simulink model "SVM_sim"  (R2018b)
settings: Solver=VariableStepAuto  StartTime=0.0  StopTime=Inf  FixedStep=T/4  RelTol=1e-3
PostLoadFcn:
  | , if any(exist('dsrtsu_mdlpostloadfcn', 'file') ~= 0), dsrtsu_mdlpostloadfcn('Execute', bdroot); end,
values from neighbouring files (symbols this model uses):
  fixed_io_gain = 175    [parameters.m]
  fixed_vclamp_gain = 1000    [parameters.m]
  fixed_vi_gain = 5800    [parameters.m]
  ioa_gain = 1    [parameters.m]
  ioa_offset = -39.67    [parameters.m]
  iob_gain = 1    [parameters.m]
  iob_offset = -40.05    [parameters.m]
  ioc_gain = 1    [parameters.m]
  ioc_offset = -39.51    [parameters.m]
  N = 500    [parameters.m]
  phi = 0    [parameters.m]
  threshold = 100    [parameters.m]
  vclamp_gain = 1    [parameters.m]
  vclamp_offset = -0.9    [parameters.m]
  via_gain = 1    [parameters.m]
  via_offset = -836.4    [parameters.m]
  vib_gain = 1    [parameters.m]
  vib_offset = -854.9    [parameters.m]
  vic_gain = 1    [parameters.m]
  vic_offset = -852.3    [parameters.m]
libraries: xbsIndex_r4 x465, rtiproclib x10, rti1202lib_adc_class1 x8, simulink x4, powerlib_meascontrol x1, rtifpgainterfacelib x1
(part 6 of 9)

== system SVM_sim/ref_generator ==
  Amp_ref : Constant  Value=5
  Constant2 : Constant  Value=2*pi/3
  Constant3 : Constant  Value=4*pi/3
  Cos : Trigonometry  Operator=cos
  Gain1 : Gain  Gain=2*pi
  Integrator : Integrator
  Multiply : Product
  Mux2 : Mux  Inputs=3
  Sum7 : Sum  Inputs=++|
  Sum8 : Sum  Inputs=++|
  f_ref : Constant  Value=50
  v_ref : Outport
  wt : Outport  Port=2
  amplitude : Outport  Port=3
  wires:
  Cos/1 -> Multiply/2
  Sum7/1 -> Mux2/2
  Sum8/1 -> Mux2/3
  Constant2/1 -> Sum7/2
  Mux2/1 -> Cos/1
  Constant3/1 -> Sum8/2
  Integrator/1 -> Sum7/1, wt/1, Sum8/1, Mux2/1
  Gain1/1 -> Integrator/1
  Multiply/1 -> v_ref/1
  f_ref/1 -> Gain1/1
  Amp_ref/1 -> amplitude/1, Multiply/1

== system SVM_sim/RTI Data/RTI Data Store ==
  RTI Data Store : Subsystem  mask(RTI_DATA_STORE){}
      mask help:
      | RTI Data Store Block. This block is used by RTI to store internal model dependent data. Deleting this block will result in data loss.
      |
      | NEVER DELETE, COPY, OR MODIFY THIS BLOCK!
      mask Help:
      | RTI Data Store Block. This block is used by RTI to store internal model dependent data. Deleting this block will result in data loss.
      | 
      | NEVER DELETE, COPY, OR MODIFY THIS BLOCK!
      mask Display: text(0.5, 0.5, ' ', 'HorizontalAlignment', 'center');

== system SVM_sim/fpga_svm/FPGA_INT_BL1 ==
  Int : Inport
  CEP1 : xbsIndex_r4/Clock Enable Probe  inherit_constraints=off  block_type=ceprobe
      settings: infoedit="Clock enable extractor.  Produces a Boolean output that mirrors the hardware clock enable associated with the input sample rate.<br><br>Hardware notes: in hardware this block costs nothing."
  Constant1 : xbsIndex_r4/Constant  const=1  gui_display_data_type=Fixed-point  arith_type=Boolean  n_bits=16  bin_pt=14  preci_type=Single  exp_width=8  frac_width=24  explicit_period=on  period=1*1e-08  equ=P=C  opselect=C  inp2=PCIN>>17  opr=+  inp1=P  carry=CIN  dbl_ovrd=off  block_type=constant
  Convert1 : xbsIndex_r4/Convert  gui_display_data_type=Fixed-point  arith_type=Unsigned  n_bits=1  bin_pt=0  float_type=Single  exp_bits=8  fraction_bits=24  quantization=Truncate  overflow=Wrap  en=off  latency=0  pipeline=off  dbl_ovrd=off  block_type=convert
  Register1 : xbsIndex_r4/Register  init=0  rst=off  en=on  dbl_ovrd=off  block_type=register
  Terminator : Terminator
  phs_interrupt : Subsystem
  usr_interrupt_00 : xbsIndex_r4/Gateway Out  inherit_from_input=off  hdl_port=on  rows=1  columns=1  UseAsDAC=off  DACChannel='1'  interface=None  automatic_assignment=on  address_offset=hex2dec('00')  intf_name=''  intf_description=''  timing_constraint=None  locs_specified=off  LOCs={}  io_standard={}  block_type=gatewayout
  tag scope: CN_SVM_sim_1_read_Interrupt_1_data_o=global
  wires:
  Constant1/1 -> CEP1/1
  CEP1/1 -> Register1/2
  Register1/1 -> usr_interrupt_00/1
  Int/1 -> Convert1/1
  Convert1/1 -> Register1/1
  usr_interrupt_00/1 -> phs_interrupt/1(data_i)
  phs_interrupt/1(data_o) -> [CN_SVM_sim_1_read_Interrupt_1_data_o], Terminator/1

== system SVM_sim/fpga_svm/FPGA_INT_BL2 ==
  Int : Inport
  CEP1 : xbsIndex_r4/Clock Enable Probe  inherit_constraints=off  block_type=ceprobe
      settings: infoedit="Clock enable extractor.  Produces a Boolean output that mirrors the hardware clock enable associated with the input sample rate.<br><br>Hardware notes: in hardware this block costs nothing."
  Constant1 : xbsIndex_r4/Constant  const=1  gui_display_data_type=Fixed-point  arith_type=Boolean  n_bits=16  bin_pt=14  preci_type=Single  exp_width=8  frac_width=24  explicit_period=on  period=1*1e-08  equ=P=C  opselect=C  inp2=PCIN>>17  opr=+  inp1=P  carry=CIN  dbl_ovrd=off  block_type=constant
  Convert1 : xbsIndex_r4/Convert  gui_display_data_type=Fixed-point  arith_type=Unsigned  n_bits=1  bin_pt=0  float_type=Single  exp_bits=8  fraction_bits=24  quantization=Truncate  overflow=Wrap  en=off  latency=0  pipeline=off  dbl_ovrd=off  block_type=convert
  Register1 : xbsIndex_r4/Register  init=0  rst=off  en=on  dbl_ovrd=off  block_type=register
  Terminator : Terminator
  phs_interrupt : Subsystem
  usr_interrupt_01 : xbsIndex_r4/Gateway Out  inherit_from_input=off  hdl_port=on  rows=1  columns=1  UseAsDAC=off  DACChannel='1'  interface=None  automatic_assignment=on  address_offset=hex2dec('00')  intf_name=''  intf_description=''  timing_constraint=None  locs_specified=off  LOCs={}  io_standard={}  block_type=gatewayout
  tag scope: CN_SVM_sim_1_read_Interrupt_2_data_o=global
  wires:
  Constant1/1 -> CEP1/1
  CEP1/1 -> Register1/2
  Register1/1 -> usr_interrupt_01/1
  Int/1 -> Convert1/1
  Convert1/1 -> Register1/1
  usr_interrupt_01/1 -> phs_interrupt/1(data_i)
  phs_interrupt/1(data_o) -> [CN_SVM_sim_1_read_Interrupt_2_data_o], Terminator/1

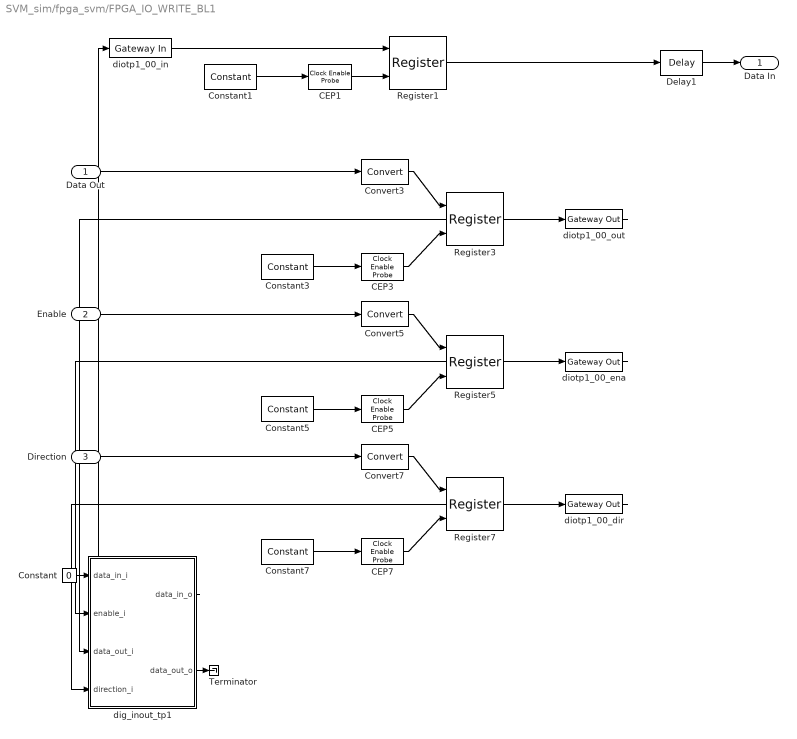
== system SVM_sim/fpga_svm/FPGA_IO_WRITE_BL1 ==
  Data Out : Inport
  Enable : Inport  Port=2
  Direction : Inport  Port=3
  CEP{1,3,5,7} (4 alike) : xbsIndex_r4/Clock Enable Probe  inherit_constraints=off  block_type=ceprobe
      settings: infoedit="Clock enable extractor.  Produces a Boolean output that mirrors the hardware clock enable associated with the input sample rate.<br><br>Hardware notes: in hardware this block costs nothing."
  Constant : Constant  Value=0
  Constant{1,3,5,7} (4 alike) : xbsIndex_r4/Constant  const=1  gui_display_data_type=Fixed-point  arith_type=Boolean  n_bits=16  bin_pt=14  preci_type=Single  exp_width=8  frac_width=24  explicit_period=on  period=1*1e-08  equ=P=C  opselect=C  inp2=PCIN>>17  opr=+  inp1=P  carry=CIN  dbl_ovrd=off  block_type=constant
  Convert3 : xbsIndex_r4/Convert  gui_display_data_type=Fixed-point  arith_type=Unsigned  n_bits=1  bin_pt=0  float_type=Single  exp_bits=8  fraction_bits=24  quantization=Truncate  overflow=Wrap  en=off  latency=0  pipeline=off  dbl_ovrd=off  block_type=convert
  Convert5 : xbsIndex_r4/Convert  gui_display_data_type=Fixed-point  arith_type=Unsigned  n_bits=1  bin_pt=0  float_type=Single  exp_bits=8  fraction_bits=24  quantization=Truncate  overflow=Wrap  en=off  latency=0  pipeline=off  dbl_ovrd=off  block_type=convert
  Convert7 : xbsIndex_r4/Convert  gui_display_data_type=Fixed-point  arith_type=Unsigned  n_bits=1  bin_pt=0  float_type=Single  exp_bits=8  fraction_bits=24  quantization=Truncate  overflow=Wrap  en=off  latency=0  pipeline=off  dbl_ovrd=off  block_type=convert
  Delay1 : xbsIndex_r4/Delay  rst=off  infoeditControl=Selection of Reset will increase slice count due to use of real FFs and instead of SRLs  en=off  latency=0  reg_retiming=off  dbl_ovrd=off  block_type=delay
  Register{1,3,5,7} (4 alike) : xbsIndex_r4/Register  init=0  rst=off  en=on  dbl_ovrd=off  block_type=register
  Terminator : Terminator
  dig_inout_tp1 : Subsystem
      mask init:
      | par = rtifpgafcnlib('GetCurrentParaValue', get_param(get(gcbh, 'parent'), 'handle'));
      | inverted_dio = str2double(par(2).Value{1});
      | vsetting = str2double(par(5).Value{1});
      | switch vsetting 
      |     case 1
      |         voltage = 3.3
      |     case 2
      |         voltage = 2.5;
      |     otherwise
      |         voltage = 5;
      | end
  diotp1_00_dir : xbsIndex_r4/Gateway Out  inherit_from_input=off  hdl_port=on  rows=1  columns=1  UseAsDAC=off  DACChannel='1'  interface=None  automatic_assignment=on  address_offset=hex2dec('00')  intf_name=''  intf_description=''  timing_constraint=None  locs_specified=off  LOCs={}  io_standard={}  block_type=gatewayout
  diotp1_00_ena : xbsIndex_r4/Gateway Out  inherit_from_input=off  hdl_port=on  rows=1  columns=1  UseAsDAC=off  DACChannel='1'  interface=None  automatic_assignment=on  address_offset=hex2dec('00')  intf_name=''  intf_description=''  timing_constraint=None  locs_specified=off  LOCs={}  io_standard={}  block_type=gatewayout
  diotp1_00_in : xbsIndex_r4/Gateway In  gui_display_data_type=Fixed-point  arith_type=Unsigned  n_bits=1  bin_pt=0  preci_type=Single  exp_width=8  frac_width=24  rows=1  columns=1  quantization="Round  (unbiased: +/- Inf)"  overflow=Saturate  period=1e-08  UseAsADC=off  ADCChannel='1'  interface=None  automatic_assignment=on  address_offset=hex2dec('00')  intf_name=''  intf_description=''  default_value=0  timing_constraint=None  locs_specified=off  LOCs={}  io_standard={}  inherit_from_input=off  hdl_port=on  dbl_ovrd=off  block_type=gatewayin
  diotp1_00_out : xbsIndex_r4/Gateway Out  inherit_from_input=off  hdl_port=on  rows=1  columns=1  UseAsDAC=off  DACChannel='1'  interface=None  automatic_assignment=on  address_offset=hex2dec('00')  intf_name=''  intf_description=''  timing_constraint=None  locs_specified=off  LOCs={}  io_standard={}  block_type=gatewayout
  Data In : Outport
  wires:
  Register1/1 -> Delay1/1
  Delay1/1 -> Data In/1
  Constant1/1 -> CEP1/1
  CEP1/1 -> Register1/2
  diotp1_00_in/1 -> Register1/1
  Constant3/1 -> CEP3/1
  CEP3/1 -> Register3/2
  Register3/1 -> diotp1_00_out/1
  Data Out/1 -> Convert3/1
  Convert3/1 -> Register3/1
  Constant5/1 -> CEP5/1
  CEP5/1 -> Register5/2
  Register5/1 -> diotp1_00_ena/1
  Enable/1 -> Convert5/1
  Convert5/1 -> Register5/1
  Constant7/1 -> CEP7/1
  CEP7/1 -> Register7/2
  Register7/1 -> diotp1_00_dir/1
  Direction/1 -> Convert7/1
  Convert7/1 -> Register7/1
  dig_inout_tp1/1(data_in_o) -> diotp1_00_in/1
  diotp1_00_out/1 -> dig_inout_tp1/3(data_out_i)
  diotp1_00_ena/1 -> dig_inout_tp1/2(enable_i)
  diotp1_00_dir/1 -> dig_inout_tp1/4(direction_i)
  Constant/1 -> dig_inout_tp1/1(data_in_i)
  dig_inout_tp1/2(data_out_o) -> Terminator/1

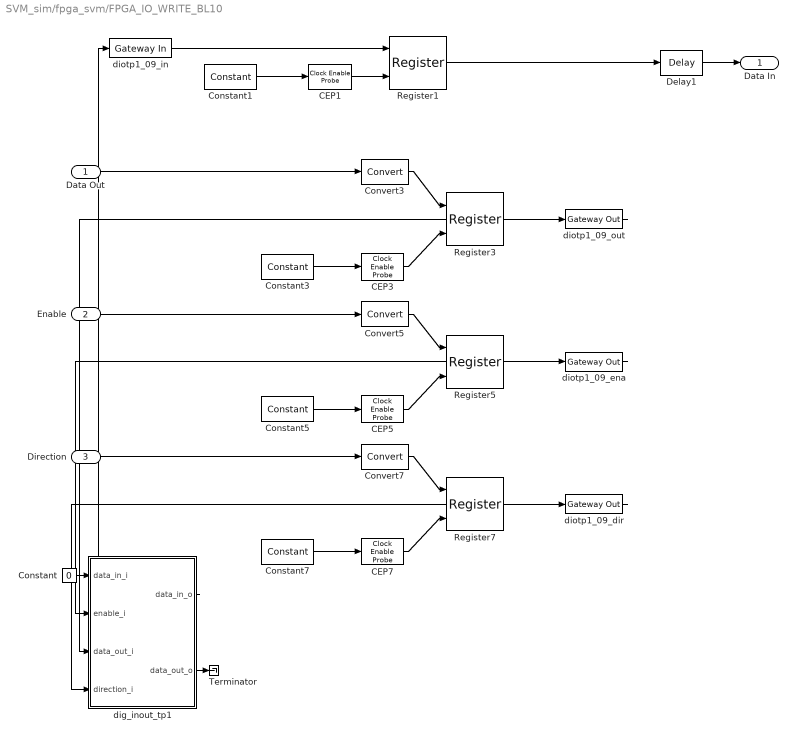
== system SVM_sim/fpga_svm/FPGA_IO_WRITE_BL10 ==
  Data Out : Inport
  Enable : Inport  Port=2
  Direction : Inport  Port=3
  CEP{1,3,5,7} (4 alike) : xbsIndex_r4/Clock Enable Probe  inherit_constraints=off  block_type=ceprobe
      settings: infoedit="Clock enable extractor.  Produces a Boolean output that mirrors the hardware clock enable associated with the input sample rate.<br><br>Hardware notes: in hardware this block costs nothing."
  Constant : Constant  Value=0
  Constant{1,3,5,7} (4 alike) : xbsIndex_r4/Constant  const=1  gui_display_data_type=Fixed-point  arith_type=Boolean  n_bits=16  bin_pt=14  preci_type=Single  exp_width=8  frac_width=24  explicit_period=on  period=1*1e-08  equ=P=C  opselect=C  inp2=PCIN>>17  opr=+  inp1=P  carry=CIN  dbl_ovrd=off  block_type=constant
  Convert3 : xbsIndex_r4/Convert  gui_display_data_type=Fixed-point  arith_type=Unsigned  n_bits=1  bin_pt=0  float_type=Single  exp_bits=8  fraction_bits=24  quantization=Truncate  overflow=Wrap  en=off  latency=0  pipeline=off  dbl_ovrd=off  block_type=convert
  Convert5 : xbsIndex_r4/Convert  gui_display_data_type=Fixed-point  arith_type=Unsigned  n_bits=1  bin_pt=0  float_type=Single  exp_bits=8  fraction_bits=24  quantization=Truncate  overflow=Wrap  en=off  latency=0  pipeline=off  dbl_ovrd=off  block_type=convert
  Convert7 : xbsIndex_r4/Convert  gui_display_data_type=Fixed-point  arith_type=Unsigned  n_bits=1  bin_pt=0  float_type=Single  exp_bits=8  fraction_bits=24  quantization=Truncate  overflow=Wrap  en=off  latency=0  pipeline=off  dbl_ovrd=off  block_type=convert
  Delay1 : xbsIndex_r4/Delay  rst=off  infoeditControl=Selection of Reset will increase slice count due to use of real FFs and instead of SRLs  en=off  latency=0  reg_retiming=off  dbl_ovrd=off  block_type=delay
  Register{1,3,5,7} (4 alike) : xbsIndex_r4/Register  init=0  rst=off  en=on  dbl_ovrd=off  block_type=register
  Terminator : Terminator
  dig_inout_tp1 : Subsystem
      mask init: same as SVM_sim/fpga_svm/FPGA_IO_WRITE_BL1/dig_inout_tp1
  diotp1_09_dir : xbsIndex_r4/Gateway Out  inherit_from_input=off  hdl_port=on  rows=1  columns=1  UseAsDAC=off  DACChannel='1'  interface=None  automatic_assignment=on  address_offset=hex2dec('00')  intf_name=''  intf_description=''  timing_constraint=None  locs_specified=off  LOCs={}  io_standard={}  block_type=gatewayout
  diotp1_09_ena : xbsIndex_r4/Gateway Out  inherit_from_input=off  hdl_port=on  rows=1  columns=1  UseAsDAC=off  DACChannel='1'  interface=None  automatic_assignment=on  address_offset=hex2dec('00')  intf_name=''  intf_description=''  timing_constraint=None  locs_specified=off  LOCs={}  io_standard={}  block_type=gatewayout
  diotp1_09_in : xbsIndex_r4/Gateway In  gui_display_data_type=Fixed-point  arith_type=Unsigned  n_bits=1  bin_pt=0  preci_type=Single  exp_width=8  frac_width=24  rows=1  columns=1  quantization="Round  (unbiased: +/- Inf)"  overflow=Saturate  period=1e-08  UseAsADC=off  ADCChannel='1'  interface=None  automatic_assignment=on  address_offset=hex2dec('00')  intf_name=''  intf_description=''  default_value=0  timing_constraint=None  locs_specified=off  LOCs={}  io_standard={}  inherit_from_input=off  hdl_port=on  dbl_ovrd=off  block_type=gatewayin
  diotp1_09_out : xbsIndex_r4/Gateway Out  inherit_from_input=off  hdl_port=on  rows=1  columns=1  UseAsDAC=off  DACChannel='1'  interface=None  automatic_assignment=on  address_offset=hex2dec('00')  intf_name=''  intf_description=''  timing_constraint=None  locs_specified=off  LOCs={}  io_standard={}  block_type=gatewayout
  Data In : Outport
  wires:
  Register1/1 -> Delay1/1
  Delay1/1 -> Data In/1
  Constant1/1 -> CEP1/1
  CEP1/1 -> Register1/2
  diotp1_09_in/1 -> Register1/1
  Constant3/1 -> CEP3/1
  CEP3/1 -> Register3/2
  Register3/1 -> diotp1_09_out/1
  Data Out/1 -> Convert3/1
  Convert3/1 -> Register3/1
  Constant5/1 -> CEP5/1
  CEP5/1 -> Register5/2
  Register5/1 -> diotp1_09_ena/1
  Enable/1 -> Convert5/1
  Convert5/1 -> Register5/1
  Constant7/1 -> CEP7/1
  CEP7/1 -> Register7/2
  Register7/1 -> diotp1_09_dir/1
  Direction/1 -> Convert7/1
  Convert7/1 -> Register7/1
  dig_inout_tp1/1(data_in_o) -> diotp1_09_in/1
  diotp1_09_out/1 -> dig_inout_tp1/3(data_out_i)
  diotp1_09_ena/1 -> dig_inout_tp1/2(enable_i)
  diotp1_09_dir/1 -> dig_inout_tp1/4(direction_i)
  Constant/1 -> dig_inout_tp1/1(data_in_i)
  dig_inout_tp1/2(data_out_o) -> Terminator/1

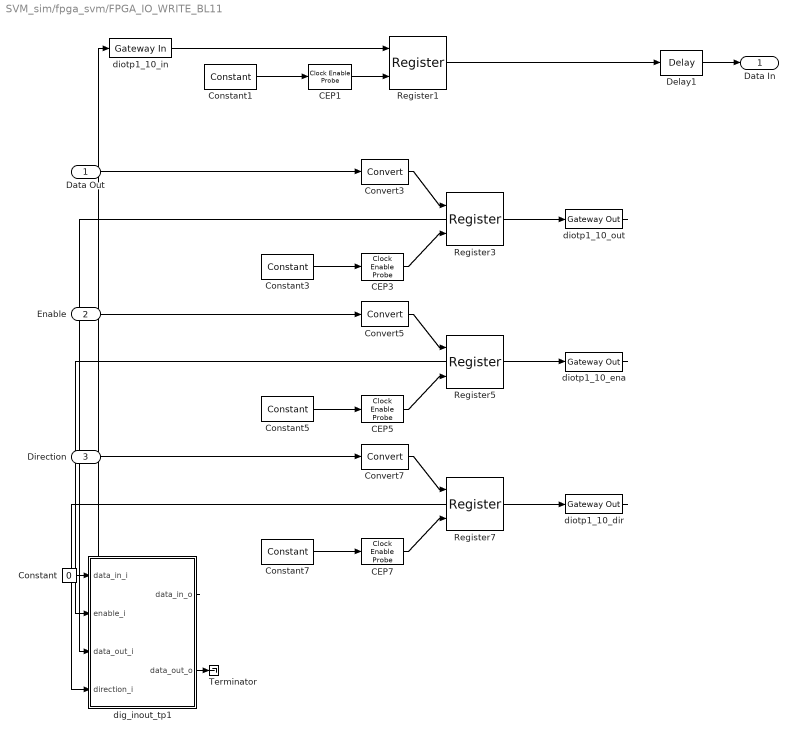
== system SVM_sim/fpga_svm/FPGA_IO_WRITE_BL11 ==
  Data Out : Inport
  Enable : Inport  Port=2
  Direction : Inport  Port=3
  CEP{1,3,5,7} (4 alike) : xbsIndex_r4/Clock Enable Probe  inherit_constraints=off  block_type=ceprobe
      settings: infoedit="Clock enable extractor.  Produces a Boolean output that mirrors the hardware clock enable associated with the input sample rate.<br><br>Hardware notes: in hardware this block costs nothing."
  Constant : Constant  Value=0
  Constant{1,3,5,7} (4 alike) : xbsIndex_r4/Constant  const=1  gui_display_data_type=Fixed-point  arith_type=Boolean  n_bits=16  bin_pt=14  preci_type=Single  exp_width=8  frac_width=24  explicit_period=on  period=1*1e-08  equ=P=C  opselect=C  inp2=PCIN>>17  opr=+  inp1=P  carry=CIN  dbl_ovrd=off  block_type=constant
  Convert3 : xbsIndex_r4/Convert  gui_display_data_type=Fixed-point  arith_type=Unsigned  n_bits=1  bin_pt=0  float_type=Single  exp_bits=8  fraction_bits=24  quantization=Truncate  overflow=Wrap  en=off  latency=0  pipeline=off  dbl_ovrd=off  block_type=convert
  Convert5 : xbsIndex_r4/Convert  gui_display_data_type=Fixed-point  arith_type=Unsigned  n_bits=1  bin_pt=0  float_type=Single  exp_bits=8  fraction_bits=24  quantization=Truncate  overflow=Wrap  en=off  latency=0  pipeline=off  dbl_ovrd=off  block_type=convert
  Convert7 : xbsIndex_r4/Convert  gui_display_data_type=Fixed-point  arith_type=Unsigned  n_bits=1  bin_pt=0  float_type=Single  exp_bits=8  fraction_bits=24  quantization=Truncate  overflow=Wrap  en=off  latency=0  pipeline=off  dbl_ovrd=off  block_type=convert
  Delay1 : xbsIndex_r4/Delay  rst=off  infoeditControl=Selection of Reset will increase slice count due to use of real FFs and instead of SRLs  en=off  latency=0  reg_retiming=off  dbl_ovrd=off  block_type=delay
  Register{1,3,5,7} (4 alike) : xbsIndex_r4/Register  init=0  rst=off  en=on  dbl_ovrd=off  block_type=register
  Terminator : Terminator
  dig_inout_tp1 : Subsystem
      mask init: same as SVM_sim/fpga_svm/FPGA_IO_WRITE_BL1/dig_inout_tp1
  diotp1_10_dir : xbsIndex_r4/Gateway Out  inherit_from_input=off  hdl_port=on  rows=1  columns=1  UseAsDAC=off  DACChannel='1'  interface=None  automatic_assignment=on  address_offset=hex2dec('00')  intf_name=''  intf_description=''  timing_constraint=None  locs_specified=off  LOCs={}  io_standard={}  block_type=gatewayout
  diotp1_10_ena : xbsIndex_r4/Gateway Out  inherit_from_input=off  hdl_port=on  rows=1  columns=1  UseAsDAC=off  DACChannel='1'  interface=None  automatic_assignment=on  address_offset=hex2dec('00')  intf_name=''  intf_description=''  timing_constraint=None  locs_specified=off  LOCs={}  io_standard={}  block_type=gatewayout
  diotp1_10_in : xbsIndex_r4/Gateway In  gui_display_data_type=Fixed-point  arith_type=Unsigned  n_bits=1  bin_pt=0  preci_type=Single  exp_width=8  frac_width=24  rows=1  columns=1  quantization="Round  (unbiased: +/- Inf)"  overflow=Saturate  period=1e-08  UseAsADC=off  ADCChannel='1'  interface=None  automatic_assignment=on  address_offset=hex2dec('00')  intf_name=''  intf_description=''  default_value=0  timing_constraint=None  locs_specified=off  LOCs={}  io_standard={}  inherit_from_input=off  hdl_port=on  dbl_ovrd=off  block_type=gatewayin
  diotp1_10_out : xbsIndex_r4/Gateway Out  inherit_from_input=off  hdl_port=on  rows=1  columns=1  UseAsDAC=off  DACChannel='1'  interface=None  automatic_assignment=on  address_offset=hex2dec('00')  intf_name=''  intf_description=''  timing_constraint=None  locs_specified=off  LOCs={}  io_standard={}  block_type=gatewayout
  Data In : Outport
  wires:
  Register1/1 -> Delay1/1
  Delay1/1 -> Data In/1
  Constant1/1 -> CEP1/1
  CEP1/1 -> Register1/2
  diotp1_10_in/1 -> Register1/1
  Constant3/1 -> CEP3/1
  CEP3/1 -> Register3/2
  Register3/1 -> diotp1_10_out/1
  Data Out/1 -> Convert3/1
  Convert3/1 -> Register3/1
  Constant5/1 -> CEP5/1
  CEP5/1 -> Register5/2
  Register5/1 -> diotp1_10_ena/1
  Enable/1 -> Convert5/1
  Convert5/1 -> Register5/1
  Constant7/1 -> CEP7/1
  CEP7/1 -> Register7/2
  Register7/1 -> diotp1_10_dir/1
  Direction/1 -> Convert7/1
  Convert7/1 -> Register7/1
  dig_inout_tp1/1(data_in_o) -> diotp1_10_in/1
  diotp1_10_out/1 -> dig_inout_tp1/3(data_out_i)
  diotp1_10_ena/1 -> dig_inout_tp1/2(enable_i)
  diotp1_10_dir/1 -> dig_inout_tp1/4(direction_i)
  Constant/1 -> dig_inout_tp1/1(data_in_i)
  dig_inout_tp1/2(data_out_o) -> Terminator/1

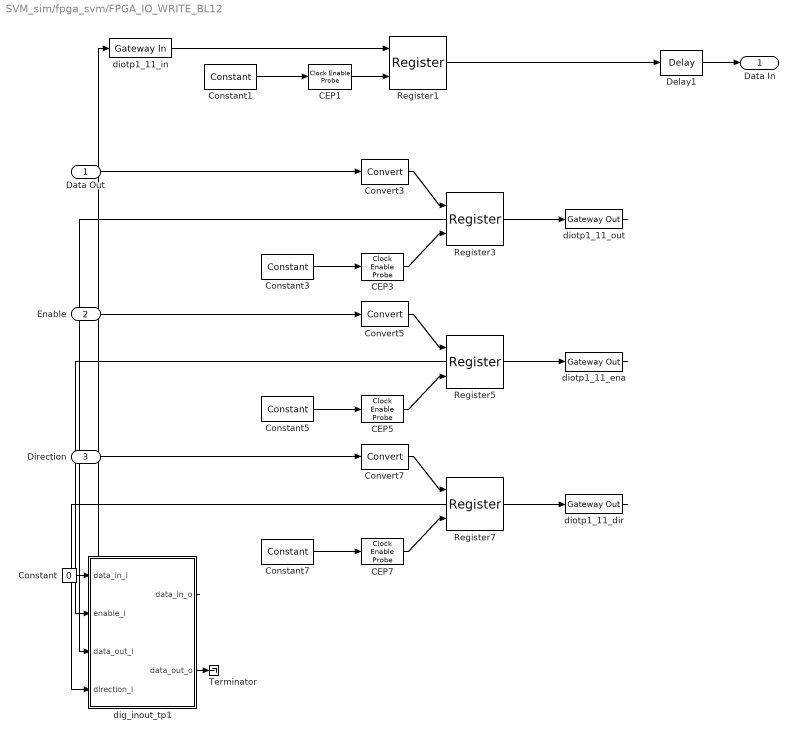
== system SVM_sim/fpga_svm/FPGA_IO_WRITE_BL12 ==
  Data Out : Inport
  Enable : Inport  Port=2
  Direction : Inport  Port=3
  CEP{1,3,5,7} (4 alike) : xbsIndex_r4/Clock Enable Probe  inherit_constraints=off  block_type=ceprobe
      settings: infoedit="Clock enable extractor.  Produces a Boolean output that mirrors the hardware clock enable associated with the input sample rate.<br><br>Hardware notes: in hardware this block costs nothing."
  Constant : Constant  Value=0
  Constant{1,3,5,7} (4 alike) : xbsIndex_r4/Constant  const=1  gui_display_data_type=Fixed-point  arith_type=Boolean  n_bits=16  bin_pt=14  preci_type=Single  exp_width=8  frac_width=24  explicit_period=on  period=1*1e-08  equ=P=C  opselect=C  inp2=PCIN>>17  opr=+  inp1=P  carry=CIN  dbl_ovrd=off  block_type=constant
  Convert3 : xbsIndex_r4/Convert  gui_display_data_type=Fixed-point  arith_type=Unsigned  n_bits=1  bin_pt=0  float_type=Single  exp_bits=8  fraction_bits=24  quantization=Truncate  overflow=Wrap  en=off  latency=0  pipeline=off  dbl_ovrd=off  block_type=convert
  Convert5 : xbsIndex_r4/Convert  gui_display_data_type=Fixed-point  arith_type=Unsigned  n_bits=1  bin_pt=0  float_type=Single  exp_bits=8  fraction_bits=24  quantization=Truncate  overflow=Wrap  en=off  latency=0  pipeline=off  dbl_ovrd=off  block_type=convert
  Convert7 : xbsIndex_r4/Convert  gui_display_data_type=Fixed-point  arith_type=Unsigned  n_bits=1  bin_pt=0  float_type=Single  exp_bits=8  fraction_bits=24  quantization=Truncate  overflow=Wrap  en=off  latency=0  pipeline=off  dbl_ovrd=off  block_type=convert
  Delay1 : xbsIndex_r4/Delay  rst=off  infoeditControl=Selection of Reset will increase slice count due to use of real FFs and instead of SRLs  en=off  latency=0  reg_retiming=off  dbl_ovrd=off  block_type=delay
  Register{1,3,5,7} (4 alike) : xbsIndex_r4/Register  init=0  rst=off  en=on  dbl_ovrd=off  block_type=register
  Terminator : Terminator
  dig_inout_tp1 : Subsystem
      mask init: same as SVM_sim/fpga_svm/FPGA_IO_WRITE_BL1/dig_inout_tp1
  diotp1_11_dir : xbsIndex_r4/Gateway Out  inherit_from_input=off  hdl_port=on  rows=1  columns=1  UseAsDAC=off  DACChannel='1'  interface=None  automatic_assignment=on  address_offset=hex2dec('00')  intf_name=''  intf_description=''  timing_constraint=None  locs_specified=off  LOCs={}  io_standard={}  block_type=gatewayout
  diotp1_11_ena : xbsIndex_r4/Gateway Out  inherit_from_input=off  hdl_port=on  rows=1  columns=1  UseAsDAC=off  DACChannel='1'  interface=None  automatic_assignment=on  address_offset=hex2dec('00')  intf_name=''  intf_description=''  timing_constraint=None  locs_specified=off  LOCs={}  io_standard={}  block_type=gatewayout
  diotp1_11_in : xbsIndex_r4/Gateway In  gui_display_data_type=Fixed-point  arith_type=Unsigned  n_bits=1  bin_pt=0  preci_type=Single  exp_width=8  frac_width=24  rows=1  columns=1  quantization="Round  (unbiased: +/- Inf)"  overflow=Saturate  period=1e-08  UseAsADC=off  ADCChannel='1'  interface=None  automatic_assignment=on  address_offset=hex2dec('00')  intf_name=''  intf_description=''  default_value=0  timing_constraint=None  locs_specified=off  LOCs={}  io_standard={}  inherit_from_input=off  hdl_port=on  dbl_ovrd=off  block_type=gatewayin
  diotp1_11_out : xbsIndex_r4/Gateway Out  inherit_from_input=off  hdl_port=on  rows=1  columns=1  UseAsDAC=off  DACChannel='1'  interface=None  automatic_assignment=on  address_offset=hex2dec('00')  intf_name=''  intf_description=''  timing_constraint=None  locs_specified=off  LOCs={}  io_standard={}  block_type=gatewayout
  Data In : Outport
  wires:
  Register1/1 -> Delay1/1
  Delay1/1 -> Data In/1
  Constant1/1 -> CEP1/1
  CEP1/1 -> Register1/2
  diotp1_11_in/1 -> Register1/1
  Constant3/1 -> CEP3/1
  CEP3/1 -> Register3/2
  Register3/1 -> diotp1_11_out/1
  Data Out/1 -> Convert3/1
  Convert3/1 -> Register3/1
  Constant5/1 -> CEP5/1
  CEP5/1 -> Register5/2
  Register5/1 -> diotp1_11_ena/1
  Enable/1 -> Convert5/1
  Convert5/1 -> Register5/1
  Constant7/1 -> CEP7/1
  CEP7/1 -> Register7/2
  Register7/1 -> diotp1_11_dir/1
  Direction/1 -> Convert7/1
  Convert7/1 -> Register7/1
  dig_inout_tp1/1(data_in_o) -> diotp1_11_in/1
  diotp1_11_out/1 -> dig_inout_tp1/3(data_out_i)
  diotp1_11_ena/1 -> dig_inout_tp1/2(enable_i)
  diotp1_11_dir/1 -> dig_inout_tp1/4(direction_i)
  Constant/1 -> dig_inout_tp1/1(data_in_i)
  dig_inout_tp1/2(data_out_o) -> Terminator/1

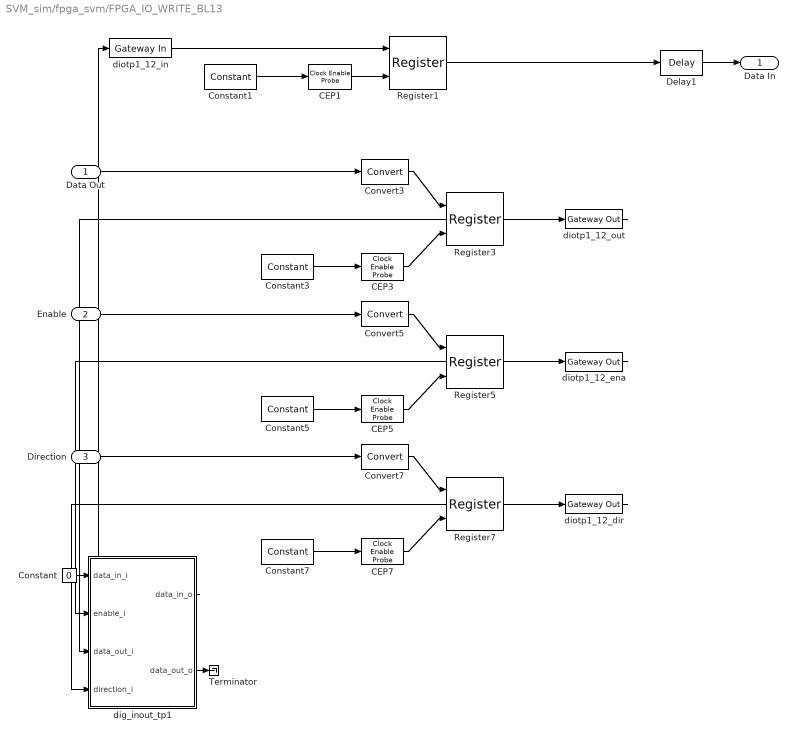
== system SVM_sim/fpga_svm/FPGA_IO_WRITE_BL13 ==
  Data Out : Inport
  Enable : Inport  Port=2
  Direction : Inport  Port=3
  CEP{1,3,5,7} (4 alike) : xbsIndex_r4/Clock Enable Probe  inherit_constraints=off  block_type=ceprobe
      settings: infoedit="Clock enable extractor.  Produces a Boolean output that mirrors the hardware clock enable associated with the input sample rate.<br><br>Hardware notes: in hardware this block costs nothing."
  Constant : Constant  Value=0
  Constant{1,3,5,7} (4 alike) : xbsIndex_r4/Constant  const=1  gui_display_data_type=Fixed-point  arith_type=Boolean  n_bits=16  bin_pt=14  preci_type=Single  exp_width=8  frac_width=24  explicit_period=on  period=1*1e-08  equ=P=C  opselect=C  inp2=PCIN>>17  opr=+  inp1=P  carry=CIN  dbl_ovrd=off  block_type=constant
  Convert3 : xbsIndex_r4/Convert  gui_display_data_type=Fixed-point  arith_type=Unsigned  n_bits=1  bin_pt=0  float_type=Single  exp_bits=8  fraction_bits=24  quantization=Truncate  overflow=Wrap  en=off  latency=0  pipeline=off  dbl_ovrd=off  block_type=convert
  Convert5 : xbsIndex_r4/Convert  gui_display_data_type=Fixed-point  arith_type=Unsigned  n_bits=1  bin_pt=0  float_type=Single  exp_bits=8  fraction_bits=24  quantization=Truncate  overflow=Wrap  en=off  latency=0  pipeline=off  dbl_ovrd=off  block_type=convert
  Convert7 : xbsIndex_r4/Convert  gui_display_data_type=Fixed-point  arith_type=Unsigned  n_bits=1  bin_pt=0  float_type=Single  exp_bits=8  fraction_bits=24  quantization=Truncate  overflow=Wrap  en=off  latency=0  pipeline=off  dbl_ovrd=off  block_type=convert
  Delay1 : xbsIndex_r4/Delay  rst=off  infoeditControl=Selection of Reset will increase slice count due to use of real FFs and instead of SRLs  en=off  latency=0  reg_retiming=off  dbl_ovrd=off  block_type=delay
  Register{1,3,5,7} (4 alike) : xbsIndex_r4/Register  init=0  rst=off  en=on  dbl_ovrd=off  block_type=register
  Terminator : Terminator
  dig_inout_tp1 : Subsystem
      mask init: same as SVM_sim/fpga_svm/FPGA_IO_WRITE_BL1/dig_inout_tp1
  diotp1_12_dir : xbsIndex_r4/Gateway Out  inherit_from_input=off  hdl_port=on  rows=1  columns=1  UseAsDAC=off  DACChannel='1'  interface=None  automatic_assignment=on  address_offset=hex2dec('00')  intf_name=''  intf_description=''  timing_constraint=None  locs_specified=off  LOCs={}  io_standard={}  block_type=gatewayout
  diotp1_12_ena : xbsIndex_r4/Gateway Out  inherit_from_input=off  hdl_port=on  rows=1  columns=1  UseAsDAC=off  DACChannel='1'  interface=None  automatic_assignment=on  address_offset=hex2dec('00')  intf_name=''  intf_description=''  timing_constraint=None  locs_specified=off  LOCs={}  io_standard={}  block_type=gatewayout
  diotp1_12_in : xbsIndex_r4/Gateway In  gui_display_data_type=Fixed-point  arith_type=Unsigned  n_bits=1  bin_pt=0  preci_type=Single  exp_width=8  frac_width=24  rows=1  columns=1  quantization="Round  (unbiased: +/- Inf)"  overflow=Saturate  period=1e-08  UseAsADC=off  ADCChannel='1'  interface=None  automatic_assignment=on  address_offset=hex2dec('00')  intf_name=''  intf_description=''  default_value=0  timing_constraint=None  locs_specified=off  LOCs={}  io_standard={}  inherit_from_input=off  hdl_port=on  dbl_ovrd=off  block_type=gatewayin
  diotp1_12_out : xbsIndex_r4/Gateway Out  inherit_from_input=off  hdl_port=on  rows=1  columns=1  UseAsDAC=off  DACChannel='1'  interface=None  automatic_assignment=on  address_offset=hex2dec('00')  intf_name=''  intf_description=''  timing_constraint=None  locs_specified=off  LOCs={}  io_standard={}  block_type=gatewayout
  Data In : Outport
  wires:
  Register1/1 -> Delay1/1
  Delay1/1 -> Data In/1
  Constant1/1 -> CEP1/1
  CEP1/1 -> Register1/2
  diotp1_12_in/1 -> Register1/1
  Constant3/1 -> CEP3/1
  CEP3/1 -> Register3/2
  Register3/1 -> diotp1_12_out/1
  Data Out/1 -> Convert3/1
  Convert3/1 -> Register3/1
  Constant5/1 -> CEP5/1
  CEP5/1 -> Register5/2
  Register5/1 -> diotp1_12_ena/1
  Enable/1 -> Convert5/1
  Convert5/1 -> Register5/1
  Constant7/1 -> CEP7/1
  CEP7/1 -> Register7/2
  Register7/1 -> diotp1_12_dir/1
  Direction/1 -> Convert7/1
  Convert7/1 -> Register7/1
  dig_inout_tp1/1(data_in_o) -> diotp1_12_in/1
  diotp1_12_out/1 -> dig_inout_tp1/3(data_out_i)
  diotp1_12_ena/1 -> dig_inout_tp1/2(enable_i)
  diotp1_12_dir/1 -> dig_inout_tp1/4(direction_i)
  Constant/1 -> dig_inout_tp1/1(data_in_i)
  dig_inout_tp1/2(data_out_o) -> Terminator/1

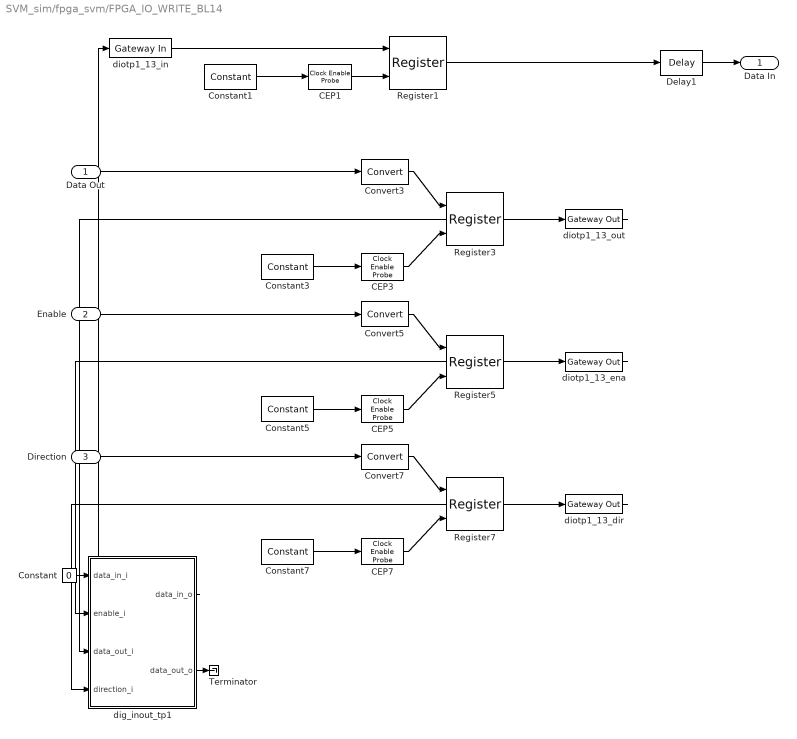
== system SVM_sim/fpga_svm/FPGA_IO_WRITE_BL14 ==
  Data Out : Inport
  Enable : Inport  Port=2
  Direction : Inport  Port=3
  CEP{1,3,5,7} (4 alike) : xbsIndex_r4/Clock Enable Probe  inherit_constraints=off  block_type=ceprobe
      settings: infoedit="Clock enable extractor.  Produces a Boolean output that mirrors the hardware clock enable associated with the input sample rate.<br><br>Hardware notes: in hardware this block costs nothing."
  Constant : Constant  Value=0
  Constant{1,3,5,7} (4 alike) : xbsIndex_r4/Constant  const=1  gui_display_data_type=Fixed-point  arith_type=Boolean  n_bits=16  bin_pt=14  preci_type=Single  exp_width=8  frac_width=24  explicit_period=on  period=1*1e-08  equ=P=C  opselect=C  inp2=PCIN>>17  opr=+  inp1=P  carry=CIN  dbl_ovrd=off  block_type=constant
  Convert3 : xbsIndex_r4/Convert  gui_display_data_type=Fixed-point  arith_type=Unsigned  n_bits=1  bin_pt=0  float_type=Single  exp_bits=8  fraction_bits=24  quantization=Truncate  overflow=Wrap  en=off  latency=0  pipeline=off  dbl_ovrd=off  block_type=convert
  Convert5 : xbsIndex_r4/Convert  gui_display_data_type=Fixed-point  arith_type=Unsigned  n_bits=1  bin_pt=0  float_type=Single  exp_bits=8  fraction_bits=24  quantization=Truncate  overflow=Wrap  en=off  latency=0  pipeline=off  dbl_ovrd=off  block_type=convert
  Convert7 : xbsIndex_r4/Convert  gui_display_data_type=Fixed-point  arith_type=Unsigned  n_bits=1  bin_pt=0  float_type=Single  exp_bits=8  fraction_bits=24  quantization=Truncate  overflow=Wrap  en=off  latency=0  pipeline=off  dbl_ovrd=off  block_type=convert
  Delay1 : xbsIndex_r4/Delay  rst=off  infoeditControl=Selection of Reset will increase slice count due to use of real FFs and instead of SRLs  en=off  latency=0  reg_retiming=off  dbl_ovrd=off  block_type=delay
  Register{1,3,5,7} (4 alike) : xbsIndex_r4/Register  init=0  rst=off  en=on  dbl_ovrd=off  block_type=register
  Terminator : Terminator
  dig_inout_tp1 : Subsystem
      mask init: same as SVM_sim/fpga_svm/FPGA_IO_WRITE_BL1/dig_inout_tp1
  diotp1_13_dir : xbsIndex_r4/Gateway Out  inherit_from_input=off  hdl_port=on  rows=1  columns=1  UseAsDAC=off  DACChannel='1'  interface=None  automatic_assignment=on  address_offset=hex2dec('00')  intf_name=''  intf_description=''  timing_constraint=None  locs_specified=off  LOCs={}  io_standard={}  block_type=gatewayout
  diotp1_13_ena : xbsIndex_r4/Gateway Out  inherit_from_input=off  hdl_port=on  rows=1  columns=1  UseAsDAC=off  DACChannel='1'  interface=None  automatic_assignment=on  address_offset=hex2dec('00')  intf_name=''  intf_description=''  timing_constraint=None  locs_specified=off  LOCs={}  io_standard={}  block_type=gatewayout
  diotp1_13_in : xbsIndex_r4/Gateway In  gui_display_data_type=Fixed-point  arith_type=Unsigned  n_bits=1  bin_pt=0  preci_type=Single  exp_width=8  frac_width=24  rows=1  columns=1  quantization="Round  (unbiased: +/- Inf)"  overflow=Saturate  period=1e-08  UseAsADC=off  ADCChannel='1'  interface=None  automatic_assignment=on  address_offset=hex2dec('00')  intf_name=''  intf_description=''  default_value=0  timing_constraint=None  locs_specified=off  LOCs={}  io_standard={}  inherit_from_input=off  hdl_port=on  dbl_ovrd=off  block_type=gatewayin
  diotp1_13_out : xbsIndex_r4/Gateway Out  inherit_from_input=off  hdl_port=on  rows=1  columns=1  UseAsDAC=off  DACChannel='1'  interface=None  automatic_assignment=on  address_offset=hex2dec('00')  intf_name=''  intf_description=''  timing_constraint=None  locs_specified=off  LOCs={}  io_standard={}  block_type=gatewayout
  Data In : Outport
  wires:
  Register1/1 -> Delay1/1
  Delay1/1 -> Data In/1
  Constant1/1 -> CEP1/1
  CEP1/1 -> Register1/2
  diotp1_13_in/1 -> Register1/1
  Constant3/1 -> CEP3/1
  CEP3/1 -> Register3/2
  Register3/1 -> diotp1_13_out/1
  Data Out/1 -> Convert3/1
  Convert3/1 -> Register3/1
  Constant5/1 -> CEP5/1
  CEP5/1 -> Register5/2
  Register5/1 -> diotp1_13_ena/1
  Enable/1 -> Convert5/1
  Convert5/1 -> Register5/1
  Constant7/1 -> CEP7/1
  CEP7/1 -> Register7/2
  Register7/1 -> diotp1_13_dir/1
  Direction/1 -> Convert7/1
  Convert7/1 -> Register7/1
  dig_inout_tp1/1(data_in_o) -> diotp1_13_in/1
  diotp1_13_out/1 -> dig_inout_tp1/3(data_out_i)
  diotp1_13_ena/1 -> dig_inout_tp1/2(enable_i)
  diotp1_13_dir/1 -> dig_inout_tp1/4(direction_i)
  Constant/1 -> dig_inout_tp1/1(data_in_i)
  dig_inout_tp1/2(data_out_o) -> Terminator/1

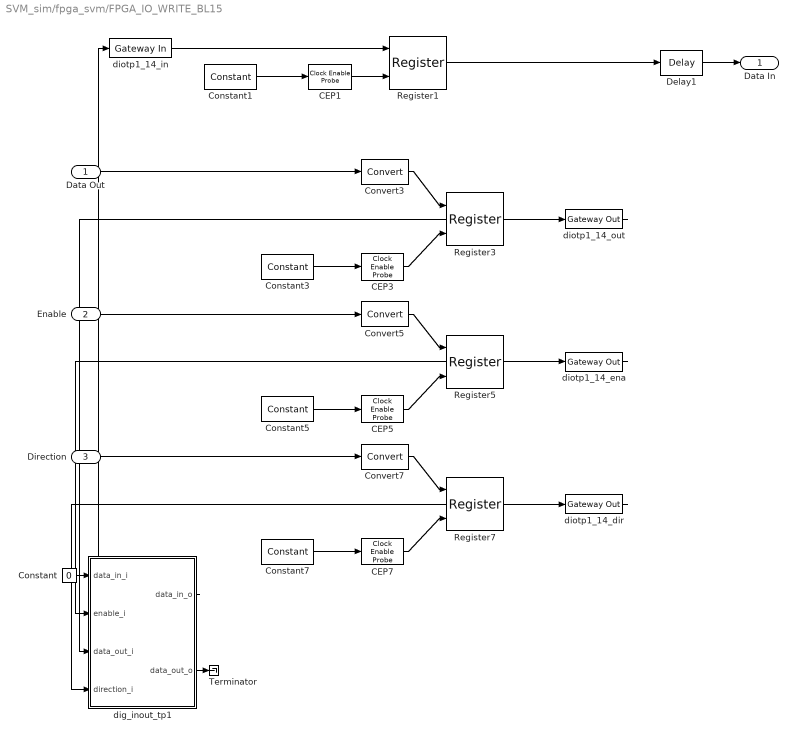
== system SVM_sim/fpga_svm/FPGA_IO_WRITE_BL15 ==
  Data Out : Inport
  Enable : Inport  Port=2
  Direction : Inport  Port=3
  CEP{1,3,5,7} (4 alike) : xbsIndex_r4/Clock Enable Probe  inherit_constraints=off  block_type=ceprobe
      settings: infoedit="Clock enable extractor.  Produces a Boolean output that mirrors the hardware clock enable associated with the input sample rate.<br><br>Hardware notes: in hardware this block costs nothing."
  Constant : Constant  Value=0
  Constant{1,3,5,7} (4 alike) : xbsIndex_r4/Constant  const=1  gui_display_data_type=Fixed-point  arith_type=Boolean  n_bits=16  bin_pt=14  preci_type=Single  exp_width=8  frac_width=24  explicit_period=on  period=1*1e-08  equ=P=C  opselect=C  inp2=PCIN>>17  opr=+  inp1=P  carry=CIN  dbl_ovrd=off  block_type=constant
  Convert3 : xbsIndex_r4/Convert  gui_display_data_type=Fixed-point  arith_type=Unsigned  n_bits=1  bin_pt=0  float_type=Single  exp_bits=8  fraction_bits=24  quantization=Truncate  overflow=Wrap  en=off  latency=0  pipeline=off  dbl_ovrd=off  block_type=convert
  Convert5 : xbsIndex_r4/Convert  gui_display_data_type=Fixed-point  arith_type=Unsigned  n_bits=1  bin_pt=0  float_type=Single  exp_bits=8  fraction_bits=24  quantization=Truncate  overflow=Wrap  en=off  latency=0  pipeline=off  dbl_ovrd=off  block_type=convert
  Convert7 : xbsIndex_r4/Convert  gui_display_data_type=Fixed-point  arith_type=Unsigned  n_bits=1  bin_pt=0  float_type=Single  exp_bits=8  fraction_bits=24  quantization=Truncate  overflow=Wrap  en=off  latency=0  pipeline=off  dbl_ovrd=off  block_type=convert
  Delay1 : xbsIndex_r4/Delay  rst=off  infoeditControl=Selection of Reset will increase slice count due to use of real FFs and instead of SRLs  en=off  latency=0  reg_retiming=off  dbl_ovrd=off  block_type=delay
  Register{1,3,5,7} (4 alike) : xbsIndex_r4/Register  init=0  rst=off  en=on  dbl_ovrd=off  block_type=register
  Terminator : Terminator
  dig_inout_tp1 : Subsystem
      mask init: same as SVM_sim/fpga_svm/FPGA_IO_WRITE_BL1/dig_inout_tp1
  diotp1_14_dir : xbsIndex_r4/Gateway Out  inherit_from_input=off  hdl_port=on  rows=1  columns=1  UseAsDAC=off  DACChannel='1'  interface=None  automatic_assignment=on  address_offset=hex2dec('00')  intf_name=''  intf_description=''  timing_constraint=None  locs_specified=off  LOCs={}  io_standard={}  block_type=gatewayout
  diotp1_14_ena : xbsIndex_r4/Gateway Out  inherit_from_input=off  hdl_port=on  rows=1  columns=1  UseAsDAC=off  DACChannel='1'  interface=None  automatic_assignment=on  address_offset=hex2dec('00')  intf_name=''  intf_description=''  timing_constraint=None  locs_specified=off  LOCs={}  io_standard={}  block_type=gatewayout
  diotp1_14_in : xbsIndex_r4/Gateway In  gui_display_data_type=Fixed-point  arith_type=Unsigned  n_bits=1  bin_pt=0  preci_type=Single  exp_width=8  frac_width=24  rows=1  columns=1  quantization="Round  (unbiased: +/- Inf)"  overflow=Saturate  period=1e-08  UseAsADC=off  ADCChannel='1'  interface=None  automatic_assignment=on  address_offset=hex2dec('00')  intf_name=''  intf_description=''  default_value=0  timing_constraint=None  locs_specified=off  LOCs={}  io_standard={}  inherit_from_input=off  hdl_port=on  dbl_ovrd=off  block_type=gatewayin
  diotp1_14_out : xbsIndex_r4/Gateway Out  inherit_from_input=off  hdl_port=on  rows=1  columns=1  UseAsDAC=off  DACChannel='1'  interface=None  automatic_assignment=on  address_offset=hex2dec('00')  intf_name=''  intf_description=''  timing_constraint=None  locs_specified=off  LOCs={}  io_standard={}  block_type=gatewayout
  Data In : Outport
  wires:
  Register1/1 -> Delay1/1
  Delay1/1 -> Data In/1
  Constant1/1 -> CEP1/1
  CEP1/1 -> Register1/2
  diotp1_14_in/1 -> Register1/1
  Constant3/1 -> CEP3/1
  CEP3/1 -> Register3/2
  Register3/1 -> diotp1_14_out/1
  Data Out/1 -> Convert3/1
  Convert3/1 -> Register3/1
  Constant5/1 -> CEP5/1
  CEP5/1 -> Register5/2
  Register5/1 -> diotp1_14_ena/1
  Enable/1 -> Convert5/1
  Convert5/1 -> Register5/1
  Constant7/1 -> CEP7/1
  CEP7/1 -> Register7/2
  Register7/1 -> diotp1_14_dir/1
  Direction/1 -> Convert7/1
  Convert7/1 -> Register7/1
  dig_inout_tp1/1(data_in_o) -> diotp1_14_in/1
  diotp1_14_out/1 -> dig_inout_tp1/3(data_out_i)
  diotp1_14_ena/1 -> dig_inout_tp1/2(enable_i)
  diotp1_14_dir/1 -> dig_inout_tp1/4(direction_i)
  Constant/1 -> dig_inout_tp1/1(data_in_i)
  dig_inout_tp1/2(data_out_o) -> Terminator/1

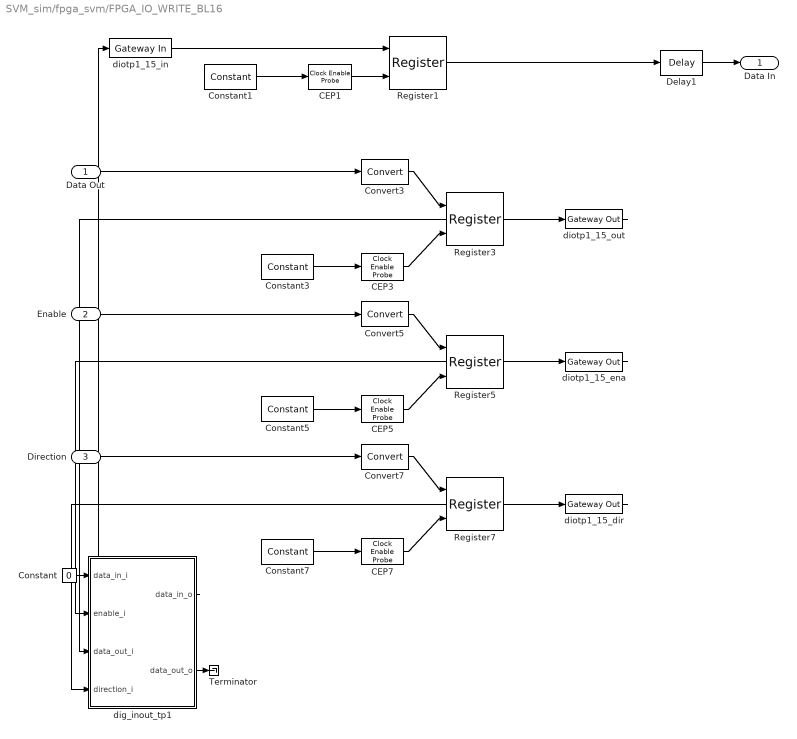
== system SVM_sim/fpga_svm/FPGA_IO_WRITE_BL16 ==
  Data Out : Inport
  Enable : Inport  Port=2
  Direction : Inport  Port=3
  CEP{1,3,5,7} (4 alike) : xbsIndex_r4/Clock Enable Probe  inherit_constraints=off  block_type=ceprobe
      settings: infoedit="Clock enable extractor.  Produces a Boolean output that mirrors the hardware clock enable associated with the input sample rate.<br><br>Hardware notes: in hardware this block costs nothing."
  Constant : Constant  Value=0
  Constant{1,3,5,7} (4 alike) : xbsIndex_r4/Constant  const=1  gui_display_data_type=Fixed-point  arith_type=Boolean  n_bits=16  bin_pt=14  preci_type=Single  exp_width=8  frac_width=24  explicit_period=on  period=1*1e-08  equ=P=C  opselect=C  inp2=PCIN>>17  opr=+  inp1=P  carry=CIN  dbl_ovrd=off  block_type=constant
  Convert3 : xbsIndex_r4/Convert  gui_display_data_type=Fixed-point  arith_type=Unsigned  n_bits=1  bin_pt=0  float_type=Single  exp_bits=8  fraction_bits=24  quantization=Truncate  overflow=Wrap  en=off  latency=0  pipeline=off  dbl_ovrd=off  block_type=convert
  Convert5 : xbsIndex_r4/Convert  gui_display_data_type=Fixed-point  arith_type=Unsigned  n_bits=1  bin_pt=0  float_type=Single  exp_bits=8  fraction_bits=24  quantization=Truncate  overflow=Wrap  en=off  latency=0  pipeline=off  dbl_ovrd=off  block_type=convert
  Convert7 : xbsIndex_r4/Convert  gui_display_data_type=Fixed-point  arith_type=Unsigned  n_bits=1  bin_pt=0  float_type=Single  exp_bits=8  fraction_bits=24  quantization=Truncate  overflow=Wrap  en=off  latency=0  pipeline=off  dbl_ovrd=off  block_type=convert
  Delay1 : xbsIndex_r4/Delay  rst=off  infoeditControl=Selection of Reset will increase slice count due to use of real FFs and instead of SRLs  en=off  latency=0  reg_retiming=off  dbl_ovrd=off  block_type=delay
  Register{1,3,5,7} (4 alike) : xbsIndex_r4/Register  init=0  rst=off  en=on  dbl_ovrd=off  block_type=register
  Terminator : Terminator
  dig_inout_tp1 : Subsystem
      mask init: same as SVM_sim/fpga_svm/FPGA_IO_WRITE_BL1/dig_inout_tp1
  diotp1_15_dir : xbsIndex_r4/Gateway Out  inherit_from_input=off  hdl_port=on  rows=1  columns=1  UseAsDAC=off  DACChannel='1'  interface=None  automatic_assignment=on  address_offset=hex2dec('00')  intf_name=''  intf_description=''  timing_constraint=None  locs_specified=off  LOCs={}  io_standard={}  block_type=gatewayout
  diotp1_15_ena : xbsIndex_r4/Gateway Out  inherit_from_input=off  hdl_port=on  rows=1  columns=1  UseAsDAC=off  DACChannel='1'  interface=None  automatic_assignment=on  address_offset=hex2dec('00')  intf_name=''  intf_description=''  timing_constraint=None  locs_specified=off  LOCs={}  io_standard={}  block_type=gatewayout
  diotp1_15_in : xbsIndex_r4/Gateway In  gui_display_data_type=Fixed-point  arith_type=Unsigned  n_bits=1  bin_pt=0  preci_type=Single  exp_width=8  frac_width=24  rows=1  columns=1  quantization="Round  (unbiased: +/- Inf)"  overflow=Saturate  period=1e-08  UseAsADC=off  ADCChannel='1'  interface=None  automatic_assignment=on  address_offset=hex2dec('00')  intf_name=''  intf_description=''  default_value=0  timing_constraint=None  locs_specified=off  LOCs={}  io_standard={}  inherit_from_input=off  hdl_port=on  dbl_ovrd=off  block_type=gatewayin
  diotp1_15_out : xbsIndex_r4/Gateway Out  inherit_from_input=off  hdl_port=on  rows=1  columns=1  UseAsDAC=off  DACChannel='1'  interface=None  automatic_assignment=on  address_offset=hex2dec('00')  intf_name=''  intf_description=''  timing_constraint=None  locs_specified=off  LOCs={}  io_standard={}  block_type=gatewayout
  Data In : Outport
  wires:
  Register1/1 -> Delay1/1
  Delay1/1 -> Data In/1
  Constant1/1 -> CEP1/1
  CEP1/1 -> Register1/2
  diotp1_15_in/1 -> Register1/1
  Constant3/1 -> CEP3/1
  CEP3/1 -> Register3/2
  Register3/1 -> diotp1_15_out/1
  Data Out/1 -> Convert3/1
  Convert3/1 -> Register3/1
  Constant5/1 -> CEP5/1
  CEP5/1 -> Register5/2
  Register5/1 -> diotp1_15_ena/1
  Enable/1 -> Convert5/1
  Convert5/1 -> Register5/1
  Constant7/1 -> CEP7/1
  CEP7/1 -> Register7/2
  Register7/1 -> diotp1_15_dir/1
  Direction/1 -> Convert7/1
  Convert7/1 -> Register7/1
  dig_inout_tp1/1(data_in_o) -> diotp1_15_in/1
  diotp1_15_out/1 -> dig_inout_tp1/3(data_out_i)
  diotp1_15_ena/1 -> dig_inout_tp1/2(enable_i)
  diotp1_15_dir/1 -> dig_inout_tp1/4(direction_i)
  Constant/1 -> dig_inout_tp1/1(data_in_i)
  dig_inout_tp1/2(data_out_o) -> Terminator/1

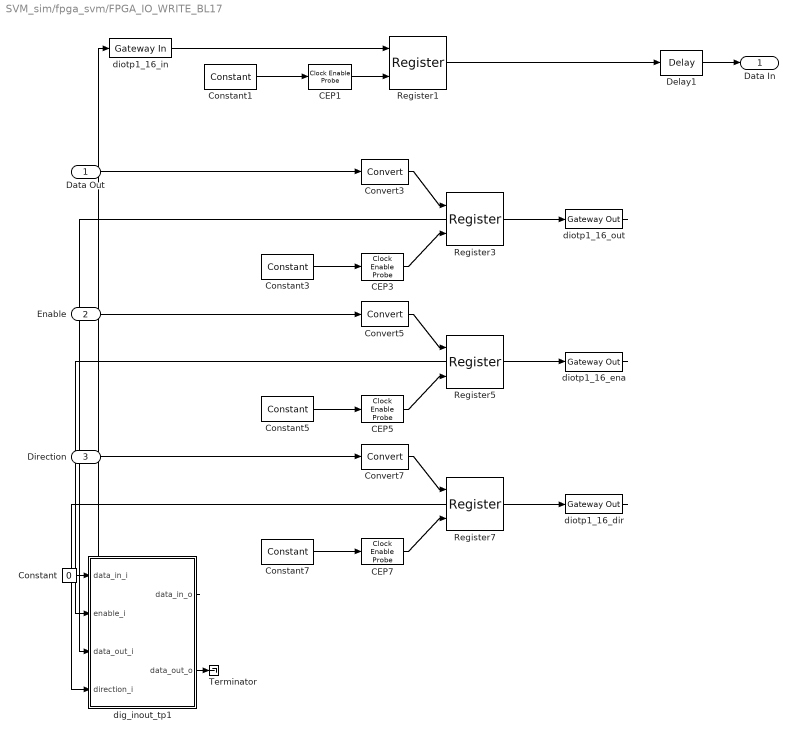
== system SVM_sim/fpga_svm/FPGA_IO_WRITE_BL17 ==
  Data Out : Inport
  Enable : Inport  Port=2
  Direction : Inport  Port=3
  CEP{1,3,5,7} (4 alike) : xbsIndex_r4/Clock Enable Probe  inherit_constraints=off  block_type=ceprobe
      settings: infoedit="Clock enable extractor.  Produces a Boolean output that mirrors the hardware clock enable associated with the input sample rate.<br><br>Hardware notes: in hardware this block costs nothing."
  Constant : Constant  Value=0
  Constant{1,3,5,7} (4 alike) : xbsIndex_r4/Constant  const=1  gui_display_data_type=Fixed-point  arith_type=Boolean  n_bits=16  bin_pt=14  preci_type=Single  exp_width=8  frac_width=24  explicit_period=on  period=1*1e-08  equ=P=C  opselect=C  inp2=PCIN>>17  opr=+  inp1=P  carry=CIN  dbl_ovrd=off  block_type=constant
  Convert3 : xbsIndex_r4/Convert  gui_display_data_type=Fixed-point  arith_type=Unsigned  n_bits=1  bin_pt=0  float_type=Single  exp_bits=8  fraction_bits=24  quantization=Truncate  overflow=Wrap  en=off  latency=0  pipeline=off  dbl_ovrd=off  block_type=convert
  Convert5 : xbsIndex_r4/Convert  gui_display_data_type=Fixed-point  arith_type=Unsigned  n_bits=1  bin_pt=0  float_type=Single  exp_bits=8  fraction_bits=24  quantization=Truncate  overflow=Wrap  en=off  latency=0  pipeline=off  dbl_ovrd=off  block_type=convert
  Convert7 : xbsIndex_r4/Convert  gui_display_data_type=Fixed-point  arith_type=Unsigned  n_bits=1  bin_pt=0  float_type=Single  exp_bits=8  fraction_bits=24  quantization=Truncate  overflow=Wrap  en=off  latency=0  pipeline=off  dbl_ovrd=off  block_type=convert
  Delay1 : xbsIndex_r4/Delay  rst=off  infoeditControl=Selection of Reset will increase slice count due to use of real FFs and instead of SRLs  en=off  latency=0  reg_retiming=off  dbl_ovrd=off  block_type=delay
  Register{1,3,5,7} (4 alike) : xbsIndex_r4/Register  init=0  rst=off  en=on  dbl_ovrd=off  block_type=register
  Terminator : Terminator
  dig_inout_tp1 : Subsystem
      mask init: same as SVM_sim/fpga_svm/FPGA_IO_WRITE_BL1/dig_inout_tp1
  diotp1_16_dir : xbsIndex_r4/Gateway Out  inherit_from_input=off  hdl_port=on  rows=1  columns=1  UseAsDAC=off  DACChannel='1'  interface=None  automatic_assignment=on  address_offset=hex2dec('00')  intf_name=''  intf_description=''  timing_constraint=None  locs_specified=off  LOCs={}  io_standard={}  block_type=gatewayout
  diotp1_16_ena : xbsIndex_r4/Gateway Out  inherit_from_input=off  hdl_port=on  rows=1  columns=1  UseAsDAC=off  DACChannel='1'  interface=None  automatic_assignment=on  address_offset=hex2dec('00')  intf_name=''  intf_description=''  timing_constraint=None  locs_specified=off  LOCs={}  io_standard={}  block_type=gatewayout
  diotp1_16_in : xbsIndex_r4/Gateway In  gui_display_data_type=Fixed-point  arith_type=Unsigned  n_bits=1  bin_pt=0  preci_type=Single  exp_width=8  frac_width=24  rows=1  columns=1  quantization="Round  (unbiased: +/- Inf)"  overflow=Saturate  period=1e-08  UseAsADC=off  ADCChannel='1'  interface=None  automatic_assignment=on  address_offset=hex2dec('00')  intf_name=''  intf_description=''  default_value=0  timing_constraint=None  locs_specified=off  LOCs={}  io_standard={}  inherit_from_input=off  hdl_port=on  dbl_ovrd=off  block_type=gatewayin
  diotp1_16_out : xbsIndex_r4/Gateway Out  inherit_from_input=off  hdl_port=on  rows=1  columns=1  UseAsDAC=off  DACChannel='1'  interface=None  automatic_assignment=on  address_offset=hex2dec('00')  intf_name=''  intf_description=''  timing_constraint=None  locs_specified=off  LOCs={}  io_standard={}  block_type=gatewayout
  Data In : Outport
  wires:
  Register1/1 -> Delay1/1
  Delay1/1 -> Data In/1
  Constant1/1 -> CEP1/1
  CEP1/1 -> Register1/2
  diotp1_16_in/1 -> Register1/1
  Constant3/1 -> CEP3/1
  CEP3/1 -> Register3/2
  Register3/1 -> diotp1_16_out/1
  Data Out/1 -> Convert3/1
  Convert3/1 -> Register3/1
  Constant5/1 -> CEP5/1
  CEP5/1 -> Register5/2
  Register5/1 -> diotp1_16_ena/1
  Enable/1 -> Convert5/1
  Convert5/1 -> Register5/1
  Constant7/1 -> CEP7/1
  CEP7/1 -> Register7/2
  Register7/1 -> diotp1_16_dir/1
  Direction/1 -> Convert7/1
  Convert7/1 -> Register7/1
  dig_inout_tp1/1(data_in_o) -> diotp1_16_in/1
  diotp1_16_out/1 -> dig_inout_tp1/3(data_out_i)
  diotp1_16_ena/1 -> dig_inout_tp1/2(enable_i)
  diotp1_16_dir/1 -> dig_inout_tp1/4(direction_i)
  Constant/1 -> dig_inout_tp1/1(data_in_i)
  dig_inout_tp1/2(data_out_o) -> Terminator/1
